simulink model "multi_quad_LED"  (Simulink 7.7)
settings: Solver=ode4  StartTime=0.0  StopTime=inf  FixedStep=sample_time_Vicon  RelTol=1e-3
InitFcn:
  | sample_time_Vicon = 0.005;
  | sample_time=0.02;
  | DeltaT = sample_time;
  | H0 = -0.1;
  | Kl = 1;
  | Omega_r = 1;
undefined symbols (not defined in the file or in its folder): DiscIntNeverNeededParam
libraries: simulink x7, dspadpt3 x1
(part 2 of 2)

== system multi_quad_LED/Vicon_Data/Raw Quad Pose from Vicon/Process Vicon Raw Data7/Flip_pi1 ==
  Angle : Inport
  Add : Sum  Inputs=-+
  Compare To Constant1 : simulink/Logic and Bit Operations/Compare To Constant  SystemSampleTime=-1  relop=>  const=pi  LogicOutDataTypeMode=uint8  ZeroCross=off
  Constant : Constant  Value=2*pi
  Data Type Duplicate : DataTypeDuplicate
  Flip_0_to_2pi : Subsystem
      mask Type: Flip zero to 2pi
      mask Description: Flips the inputs into the range zero to +2pi
      mask Help: Flips the inputs into the range zero to +2pi
      mask Display: disp('Flip_0_2pi')
  Switch : Switch  Criteria=u2 ~= 0
  Angle_Flip : Outport
  wires:
  Angle/1 -> Flip_0_to_2pi/1(Angle), Data Type Duplicate/2
  Flip_0_to_2pi/1(Angle_Flip) -> Switch/3, Compare To Constant1/1, Add/2
  Compare To Constant1/1 -> Switch/2
  Constant/1 -> Add/1
  Add/1 -> Switch/1
  Switch/1 -> Angle_Flip/1, Data Type Duplicate/1

== system multi_quad_LED/Vicon_Data/Raw Quad Pose from Vicon/Process Vicon Raw Data1/Flip_pi1/Flip_0_to_2pi ==
  Angle : Inport
  Add : Sum
  Compare To Constant1 : simulink/Logic and Bit Operations/Compare To Constant  SystemSampleTime=-1  relop=<  const=0  LogicOutDataTypeMode=uint8  ZeroCross=off
  Constant : Constant  Value=2*pi
  Data Type Duplicate : DataTypeDuplicate
  Flip_2pi : Subsystem
      mask Type: Flip -2pi to 2pi
      mask Description: Flips the inputs into the range -2pi to +2pi
      mask Help: Flips the inputs into the range -2pi to +2pi
      mask Display: disp('Flip_2pi')
  Switch : Switch  Criteria=u2 ~= 0
  Angle_Flip : Outport
  wires:
  Flip_2pi/1(Angle_Flip) -> Compare To Constant1/1, Add/2, Switch/3
  Compare To Constant1/1 -> Switch/2
  Constant/1 -> Add/1
  Add/1 -> Switch/1
  Angle/1 -> Flip_2pi/1(Angle), Data Type Duplicate/2
  Switch/1 -> Angle_Flip/1, Data Type Duplicate/1

== system multi_quad_LED/Vicon_Data/Raw Quad Pose from Vicon/Process Vicon Raw Data6/Flip_pi1/Flip_0_to_2pi ==
  Angle : Inport
  Add : Sum
  Compare To Constant1 : simulink/Logic and Bit Operations/Compare To Constant  SystemSampleTime=-1  relop=<  const=0  LogicOutDataTypeMode=uint8  ZeroCross=off
  Constant : Constant  Value=2*pi
  Data Type Duplicate : DataTypeDuplicate
  Flip_2pi : Subsystem
      mask Type: Flip -2pi to 2pi
      mask Description: Flips the inputs into the range -2pi to +2pi
      mask Help: Flips the inputs into the range -2pi to +2pi
      mask Display: disp('Flip_2pi')
  Switch : Switch  Criteria=u2 ~= 0
  Angle_Flip : Outport
  wires:
  Switch/1 -> Data Type Duplicate/1, Angle_Flip/1
  Angle/1 -> Data Type Duplicate/2, Flip_2pi/1(Angle)
  Add/1 -> Switch/1
  Constant/1 -> Add/1
  Compare To Constant1/1 -> Switch/2
  Flip_2pi/1(Angle_Flip) -> Switch/3, Add/2, Compare To Constant1/1

== system multi_quad_LED/Vicon_Data/Raw Quad Pose from Vicon/Process Vicon Raw Data7/Flip_pi1/Flip_0_to_2pi ==
  Angle : Inport
  Add : Sum
  Compare To Constant1 : simulink/Logic and Bit Operations/Compare To Constant  SystemSampleTime=-1  relop=<  const=0  LogicOutDataTypeMode=uint8  ZeroCross=off
  Constant : Constant  Value=2*pi
  Data Type Duplicate : DataTypeDuplicate
  Flip_2pi : Subsystem
      mask Type: Flip -2pi to 2pi
      mask Description: Flips the inputs into the range -2pi to +2pi
      mask Help: Flips the inputs into the range -2pi to +2pi
      mask Display: disp('Flip_2pi')
  Switch : Switch  Criteria=u2 ~= 0
  Angle_Flip : Outport
  wires:
  Flip_2pi/1(Angle_Flip) -> Compare To Constant1/1, Add/2, Switch/3
  Compare To Constant1/1 -> Switch/2
  Constant/1 -> Add/1
  Add/1 -> Switch/1
  Angle/1 -> Flip_2pi/1(Angle), Data Type Duplicate/2
  Switch/1 -> Angle_Flip/1, Data Type Duplicate/1

== system multi_quad_LED/Vicon_Data/Raw Quad Pose from Vicon/Process Vicon Raw Data1/Flip_pi1/Flip_0_to_2pi/Flip_2pi ==
  Angle : Inport
  Bias : Bias  Bias=-2*pi
  Constant : Constant  Value=2*pi
  Data Type Duplicate : DataTypeDuplicate
  Modulo : Math  Operator=mod  SaturateOnIntegerOverflow=on
  Sign1 : Signum
  Switch : Switch
  Angle_Flip : Outport
  wires:
  Angle/1 -> Modulo/1, Sign1/1, Data Type Duplicate/1
  Constant/1 -> Modulo/2
  Modulo/1 -> Bias/1, Switch/1
  Sign1/1 -> Switch/2
  Bias/1 -> Switch/3
  Switch/1 -> Angle_Flip/1, Data Type Duplicate/2

== system multi_quad_LED/Vicon_Data/Raw Quad Pose from Vicon/Process Vicon Raw Data6/Flip_pi1/Flip_0_to_2pi/Flip_2pi ==
  Angle : Inport
  Bias : Bias  Bias=-2*pi
  Constant : Constant  Value=2*pi
  Data Type Duplicate : DataTypeDuplicate
  Modulo : Math  Operator=mod  SaturateOnIntegerOverflow=on
  Sign1 : Signum
  Switch : Switch
  Angle_Flip : Outport
  wires:
  Switch/1 -> Data Type Duplicate/2, Angle_Flip/1
  Bias/1 -> Switch/3
  Sign1/1 -> Switch/2
  Modulo/1 -> Switch/1, Bias/1
  Constant/1 -> Modulo/2
  Angle/1 -> Data Type Duplicate/1, Sign1/1, Modulo/1

== system multi_quad_LED/Vicon_Data/Raw Quad Pose from Vicon/Process Vicon Raw Data7/Flip_pi1/Flip_0_to_2pi/Flip_2pi ==
  Angle : Inport
  Bias : Bias  Bias=-2*pi
  Constant : Constant  Value=2*pi
  Data Type Duplicate : DataTypeDuplicate
  Modulo : Math  Operator=mod  SaturateOnIntegerOverflow=on
  Sign1 : Signum
  Switch : Switch
  Angle_Flip : Outport
  wires:
  Angle/1 -> Modulo/1, Sign1/1, Data Type Duplicate/1
  Constant/1 -> Modulo/2
  Modulo/1 -> Bias/1, Switch/1
  Sign1/1 -> Switch/2
  Bias/1 -> Switch/3
  Switch/1 -> Angle_Flip/1, Data Type Duplicate/2

== matlab function Planning/Yaw Controller/MATLAB Function ==
  data: u input double; y output double
function y = fcn(u)
%#codegen
y = u;
if y > pi    
    y = y - 2*pi;
elseif y < -pi
        y = y + 2*pi;
end

== stateflow chart Planning/Trajectory Logic/UAV SF ==
  state Landing
    state Descending
      en:PosDesired = Pos; PWM = 1600;
      du:PosDesired[2] = (0 - PosDesired[2])*1*DeltaT + PosDesired[2] ;
    state CutThrottle
      du:HoverThrottle = (-0.95 - HoverThrottle)*2*DeltaT + HoverThrottle ;
    (default) -> Descending
    Descending -> CutThrottle : [Pos[2] > -0.2]
  state Airborne
    state TakeOff
      du:HoverThrottle = (H0 - HoverThrottle)*2*DeltaT + HoverThrottle ;
    state PreGrasp
      en:
      PosDesired[0] = ObjPos[0]-2.5*cos(ObjPos[3]);
      PosDesired[1] = ObjPos[1] -2.5*sin(ObjPos[3]);PosDesired[2] = ObjPos[2]-0.3;
      PWM = 1600;
    state Hover
    state GraspObj
      state Grasp
        en:PWM = 900;
        PosDesired[2] = Pos[2];
      state AboveObjPoint15CM
      state AboveObjPoint15CMHover
      state Descend
        en:PosDesired[2] = ObjPos[2] ;
      state Ascend
        en:PosDesired[2] = ObjPos[2] - 0.5;
      state PreGrasp1
        en:
        PosDesired[0] = ObjPos[0]-2.5*cos(ObjPos[3]);
        PosDesired[1] = ObjPos[1] -2.5*sin(ObjPos[3]);
        PosDesired[2] = ObjPos[2]-0.3;
        PosDesired[3] = ObjPos[3];
      AboveObjPoint15CM -> AboveObjPoint15CMHover : after(6,sec)
          | {PosDesired = ObjPos;PosDesired[2] = ObjPos[2] - 0.15;}
      Grasp -> Ascend : after(1,sec)
      Descend -> Grasp : [(ObjPos[2] - Pos[2]) < 0.01]
      AboveObjPoint15CMHover -> Descend : [PerchError < 0.01]
      (default) -> AboveObjPoint15CM : {PosDesired = ObjPos;PosDesired[2] = ObjPos[2] - 0.15;}
    state Home
      en:
      PosDesired[0] = -1;
      PosDesired[1] = 2;
      PosDesired[2] = -1.3;
      PosDesired[3] = ObjPos[3];
      PWM = 1600;
    state DropPoint
      en:
      PosDesired[0] = -1;PosDesired[1] = 2;
      PosDesired[2] = -0.8;PosDesired[3] = ObjPos[3];
    state LandingPoint
      en:
      PosDesired[0] = 0;
    state Drop
      en:
      PWM = 1600;
    (default) -> TakeOff : {PosDesired = Pos;  PosDesired[2] = -1;}
    TakeOff -> Hover : after(2,sec)
        | {PosDesired = Pos;}
    PreGrasp -> GraspObj : after(3,sec)
    Hover -> Home : after(2,sec)
    Home -> PreGrasp : after(2,sec)
    DropPoint -> Drop : after(8,sec)
    Drop -> LandingPoint : after(3,sec)
    Ascend -> DropPoint : after(6,sec)
  (default) -> Landing : {HoverThrottle = -0.9;}
  Airborne -> Landing : [RC[6] < -0.5]
  Landing -> Airborne : [RC[6] > 0.5]
  data: PosDesired output double size=4; HoverThrottle output double size=1; Mode output uint8 size=3; RC input double size=8; Pos input double size=4; ObjPos input double size=4; DeltaT parameter double size=1; H0 parameter double size=1; Kl parameter double size=1; VelCmd local double size=2 =0; PWM output double; PerchError input double
